simulink model "SSplHint4"  (Simulink 4.00)
settings: Solver=FixedStepDiscrete  SolverMode=SingleTasking  StartTime=0.0  StopTime=50.0  RelTol=1e-3
libraries: dspbdsp2 x15, dspsrcs2 x1
settings Model: LastModifiedBy=igors  LimitDataPoints=off  ExtModeTrigMode=oneshot  ExtModeArmWhenConnect=off

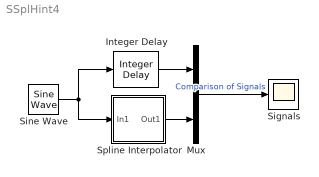
== system SSplHint4 ==
  Integer Delay : dspbdsp2/Integer Delay  delay=2  ic=0  frame=off  df=on  numChans=1
  Mux : Mux  Inputs=2
  Signals : Scope
      settings: TickLabels=on  TimeRange=auto  YMin=-1.2  YMax=1.2  SaveToWorkspace=off  SaveName=ScopeData  DataFormat=Array  LimitDataPoints=on  MaxDataPoints=5000
  Sine Wave : dspsrcs2/Sine Wave  Amplitude=1  Frequency=0.2  Phase=0  SampleMode=Discrete  OutComplex=Real  CompMethod=Trigonometric Fcn  SampleTime=1  SamplesPerFrame=1  ResetState=Restart at time zero
  Spline Interpolator : Subsystem  Description=Hermite Kub 4
      settings: RTWFcnNameOpts=Auto  RTWFileNameOpts=Auto
  wires:
  Sine Wave/1 -> Spline Interpolator/1(In1), Integer Delay/1
  Spline Interpolator/1(Out1) -> Mux/2
  Mux/1 -> Signals/1  "Comparison of Signals"
  Integer Delay/1 -> Mux/1

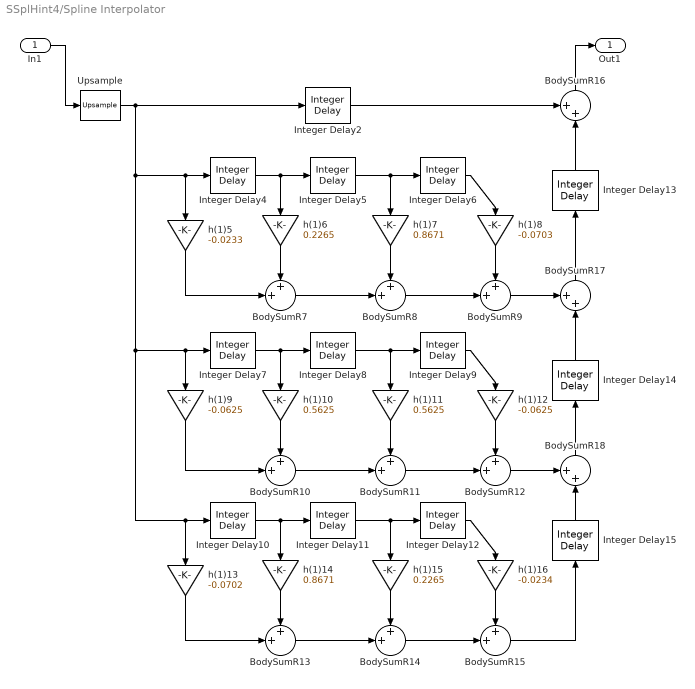
== system SSplHint4/Spline Interpolator ==
  In1 : Inport  Port=1  LatchInput=off
  BodySumR{7..15} (9 alike) : Sum  Inputs=++|  SaturateOnIntegerOverflow=on
  BodySumR16 : Sum  Orientation=up  Inputs=++|  SaturateOnIntegerOverflow=on
  BodySumR17 : Sum  Orientation=up  Inputs=++|  SaturateOnIntegerOverflow=on
  BodySumR18 : Sum  Orientation=up  Inputs=++|  SaturateOnIntegerOverflow=on
  Integer Delay{4..12} (9 alike) : dspbdsp2/Integer Delay  delay=4  ic=0  frame=off  df=on  numChans=1
  Integer Delay13 : dspbdsp2/Integer Delay  Orientation=up  delay=1  ic=0  frame=off  df=on  numChans=1
  Integer Delay14 : dspbdsp2/Integer Delay  Orientation=up  delay=1  ic=0  frame=off  df=on  numChans=1
  Integer Delay15 : dspbdsp2/Integer Delay  Orientation=up  delay=1  ic=0  frame=off  df=on  numChans=1
  Integer Delay2 : dspbdsp2/Integer Delay  delay=8  ic=0  frame=off  df=on  numChans=1
  Upsample : dspbdsp2/Upsample  N=4  phase=0  ic=0  frame=off  nchans=1  mode=Maintain input frame size
  h(1)10 : Gain  Orientation=down  Gain=0.5625  Multiplication=Element-wise(K.*u)  SaturateOnIntegerOverflow=on
  h(1)11 : Gain  Orientation=down  Gain=0.5625  Multiplication=Element-wise(K.*u)  SaturateOnIntegerOverflow=on
  h(1)12 : Gain  Orientation=down  Gain=-0.0625  Multiplication=Element-wise(K.*u)  SaturateOnIntegerOverflow=on
  h(1)13 : Gain  Orientation=down  Gain=-0.0702  Multiplication=Element-wise(K.*u)  SaturateOnIntegerOverflow=on
  h(1)14 : Gain  Orientation=down  Gain=0.8671  Multiplication=Element-wise(K.*u)  SaturateOnIntegerOverflow=on
  h(1)15 : Gain  Orientation=down  Gain=0.2265  Multiplication=Element-wise(K.*u)  SaturateOnIntegerOverflow=on
  h(1)16 : Gain  Orientation=down  Gain=-0.0234  Multiplication=Element-wise(K.*u)  SaturateOnIntegerOverflow=on
  h(1)5 : Gain  Orientation=down  Gain=-0.0233  Multiplication=Element-wise(K.*u)  SaturateOnIntegerOverflow=on
  h(1)6 : Gain  Orientation=down  Gain=0.2265  Multiplication=Element-wise(K.*u)  SaturateOnIntegerOverflow=on
  h(1)7 : Gain  Orientation=down  Gain=0.8671  Multiplication=Element-wise(K.*u)  SaturateOnIntegerOverflow=on
  h(1)8 : Gain  Orientation=down  Gain=-0.0703  Multiplication=Element-wise(K.*u)  SaturateOnIntegerOverflow=on
  h(1)9 : Gain  Orientation=down  Gain=-0.0625  Multiplication=Element-wise(K.*u)  SaturateOnIntegerOverflow=on
  Out1 : Outport  Port=1
  wires:
  In1/1 -> Upsample/1
  Upsample/1 -> Integer Delay4/1, h(1)5/1, Integer Delay10/1, h(1)13/1, Integer Delay7/1, h(1)9/1, Integer Delay2/1
  BodySumR16/1 -> Out1/1
  Integer Delay4/1 -> Integer Delay5/1, h(1)6/1
  Integer Delay5/1 -> Integer Delay6/1, h(1)7/1
  Integer Delay6/1 -> h(1)8/1
  h(1)5/1 -> BodySumR7/2
  h(1)6/1 -> BodySumR7/1
  h(1)8/1 -> BodySumR9/1
  BodySumR7/1 -> BodySumR8/2
  BodySumR8/1 -> BodySumR9/2
  Integer Delay7/1 -> Integer Delay8/1, h(1)10/1
  Integer Delay8/1 -> Integer Delay9/1, h(1)11/1
  Integer Delay9/1 -> h(1)12/1
  h(1)9/1 -> BodySumR10/2
  h(1)10/1 -> BodySumR10/1
  h(1)11/1 -> BodySumR11/1
  h(1)12/1 -> BodySumR12/1
  BodySumR10/1 -> BodySumR11/2
  BodySumR11/1 -> BodySumR12/2
  Integer Delay10/1 -> Integer Delay11/1, h(1)14/1
  Integer Delay11/1 -> Integer Delay12/1, h(1)15/1
  Integer Delay12/1 -> h(1)16/1
  h(1)13/1 -> BodySumR13/2
  h(1)14/1 -> BodySumR13/1
  h(1)15/1 -> BodySumR14/1
  h(1)16/1 -> BodySumR15/1
  BodySumR13/1 -> BodySumR14/2
  BodySumR14/1 -> BodySumR15/2
  BodySumR12/1 -> BodySumR18/1
  BodySumR9/1 -> BodySumR17/1
  BodySumR18/1 -> Integer Delay14/1
  Integer Delay14/1 -> BodySumR17/2
  Integer Delay15/1 -> BodySumR18/2
  BodySumR15/1 -> Integer Delay15/1
  BodySumR17/1 -> Integer Delay13/1
  Integer Delay13/1 -> BodySumR16/2
  Integer Delay2/1 -> BodySumR16/1
  h(1)7/1 -> BodySumR8/1
